simulink library "gm_dvbs2_stream_lib"  (R2025a)
settings: Solver=VariableStepAuto  StartTime=0.0  StopTime=10.0  RelTol=1e-3
undefined symbols (not defined in the file or in its folder): AXI4, Fs, gcbh, ip, Lite, soc
libraries: axiinterfacelib x6, xilinxsocsdrlib_internal x1, socsharedlib_internal x1
settings Model: Creator=daniel  LastModifiedBy=daniel

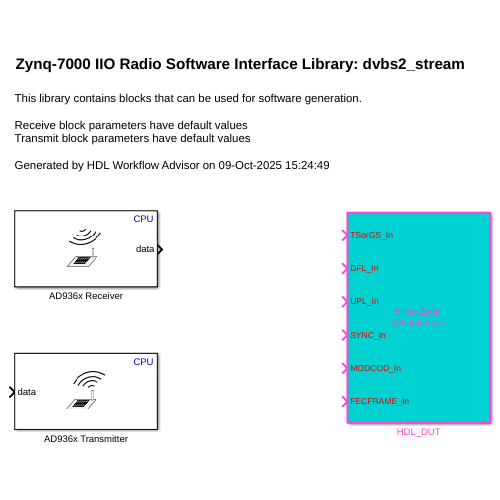
[thumbnail: Simulink's stored preview of the top-level diagram]
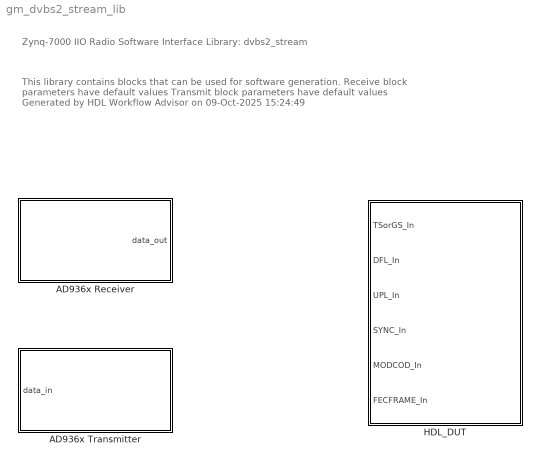
== system gm_dvbs2_stream_lib ==
  note: Zynq-7000 IIO Radio Software Interface Library: dvbs2_stream
  note: This library contains blocks that can be used for software generation.
      |
      | Receive block parameters have default values
      | Transmit block parameters have default values
      |
      | Generated by HDL Workflow Advisor on 09-Oct-2025 15:24:49
  AD936x Receiver : Subsystem  InitFcn=soc.blkcb.ad936xReadCb('InitFcn',gcbh);  mask(AD936x Data Read){SimulationInput=Zeros, IPAddress=192.168.3.2, CenterFrequencySource=Dialog, CenterFrequency=2400000000, GainSource=Dialog, Gain=10, BasebandSampleRate=1000000, EnableChannel1=on, EnableChannel2=off, OutputDataTypeStr=int16 (complex), SamplesPerFrame=20000, OverflowOutputPort=off, EnableBurstMode=off, NumFramesInBurst=2, UseCustomFilter=off, filtCoefficientSize=128, filtCoefficients=[-192 82 85 -215 228 -102 -110 290 -318 145 160 -426 471 -215 -238 633 -697 318 349 -923 1009 -457 -498 1309 -1423 640 693 -1812 1959 -876 -945 2458 -2647 1180 1268 -3290 3534 -1572 -1688 4375 -4698 2091 2247 -5836 6284 -2807 -3031 7918 -8588 3870 4225 -11182 12324 -5662 -6330 17255 -19735 9507 11312 -33568 43355 -25227 -42139 305542 305542 -42139 -25227 43355 -33568 11312 9507 -19735 17255 -6330 -5662 12324 -11182 4225 3870 -8588 7918 -3031 -2807 6284 -5836 2247 2091 -4698 4375 -1688 -1572 3534 -3290 1268 1180 -2647 2458 -945 -876 1959 -1812 693 640 -1423 1309 -498 -457 1009 -923 349 318 -697 633 -238 -215 471 -426 160 145 -318 290 -110 -102 228 -215 85 82 -192], filtDecimInterpFactor=4, filtGain=-12, filtPathRates=[737280000 11520000 3840000 1920000 960000 240000], filtRFBandwidth=18e6, filterConfigStruct=struct(), BypassUserLogic=off, EnableQuadratureCorrection=on, EnableRFDCCorrection=on, EnableBasebandDCCorrection=on, OverrideSampleTime=off, SampleTime=0.02, DataTimeout=Inf, BISTLoopbackMode=Disabled, BISTToneInject=Disabled, BISTSignalGen=PRBS, BISTToneFreq=Fs/32, BISTToneLevel=0}
      mask prompts: SimulationInput "Simulation input:"; IPAddress "Radio IP address:"; CenterFrequencySource "Source of center frequency:"; CenterFrequency "Center frequency (Hz):"; GainSource "Source of gain:"; Gain "Gain (dB):"; BasebandSampleRate "Baseband sample rate (Hz):"; EnableChannel1 "Enable Channel 1"; EnableChannel2 "Enable Channel 2"; OutputDataTypeStr "Output data type:"; SamplesPerFrame "Sample per frame:"; OverflowOutputPort "Enable output port for overflow indicator"; EnableBurstMode "Enable burst mode"; NumFramesInBurst "Frames in burst:"; UseCustomFilter "Use custom filter"; filtCoefficientSize "FIR coefficients size:"; filtCoefficients "FIR coefficients :"; filtDecimInterpFactor "FIR decimation/interpolation factor:"; filtGain "FIR gain (dB):"; filtPathRates "Filter path rates (Hz):"; filtRFBandwidth "Analog filter cutoff (Hz):"; filterConfigStruct "Filter config structure:"; BypassUserLogic "Bypass user logic"; EnableQuadratureCorrection "Enable quadrature correction"; EnableRFDCCorrection "Enable RF DC correction"; EnableBasebandDCCorrection "Enable baseband DC correction"; OverrideSampleTime "Override automatic sample time"; SampleTime "Sample time:"; DataTimeout "Data timeout (sec):"; BISTLoopbackMode "Loopback:"; BISTToneInject "Test signal injection:"; BISTSignalGen "Signal generator mode:"; BISTToneFreq "Tone frequency (Hz):"; BISTToneLevel "Tone level (dB):"
      mask help: soc:sdr:AD936xReadMaskText
      mask init:
      | soc.blkcb.ad936xReadCb('MaskInitFcn', gcbh);
      mask Help: helpview('soc', 'xilinxsoc_ad936x_data_read')
      mask TypeOptions SimulationInput: No data (configuration only) | Zeros | From connected IO
      mask Callback SimulationInput: soc.blkcb.ad936xReadCb('MaskParamCb',gcbh,'SimulationInput');
      mask TypeOptions IPAddress: Source Variant/From Connected IO/AD936x Receiver/IPAddress
      mask TypeOptions CenterFrequencySource: Source Variant/From Connected IO/AD936x Receiver/CenterFrequencySource | Source Variant/No Data/AD936x Receiver Config/CenterFrequencySource | Source Variant/Zeros/SimCodegen Variant/CODEGEN/AD936x Receiver/CenterFrequencySource
      mask Callback CenterFrequencySource: soc.blkcb.ad936xReadCb('MaskParamCb',gcbh,'CenterFrequencySource');
      mask TypeOptions CenterFrequency: Source Variant/From Connected IO/AD936x Receiver/CenterFrequency | Source Variant/No Data/AD936x Receiver Config/CenterFrequency | Source Variant/Zeros/SimCodegen Variant/CODEGEN/AD936x Receiver/CenterFrequency
      mask TypeOptions GainSource: Source Variant/From Connected IO/AD936x Receiver/GainSourceBlock | Source Variant/No Data/AD936x Receiver Config/GainSourceBlock | Source Variant/Zeros/SimCodegen Variant/CODEGEN/AD936x Receiver/GainSourceBlock
      mask Callback GainSource: soc.blkcb.ad936xReadCb('MaskParamCb',gcbh,'GainSource');
      mask TypeOptions Gain: Source Variant/From Connected IO/AD936x Receiver/Gain | Source Variant/No Data/AD936x Receiver Config/Gain | Source Variant/Zeros/SimCodegen Variant/CODEGEN/AD936x Receiver/Gain
      mask TypeOptions BasebandSampleRate: Source Variant/From Connected IO/AD936x Receiver/BasebandSampleRate | Source Variant/No Data/AD936x Receiver Config/BasebandSampleRate | Source Variant/Zeros/SimCodegen Variant/CODEGEN/AD936x Receiver/BasebandSampleRate
      mask TypeOptions OutputDataTypeStr: int16 (complex) | single (complex) | double (complex)
      mask TypeOptions OverflowOutputPort: Source Variant/From Connected IO/AD936x Receiver/OverflowOutputPort | Source Variant/Zeros/SimCodegen Variant/CODEGEN/AD936x Receiver/OverflowOutputPort
      mask TypeOptions EnableBurstMode: Source Variant/From Connected IO/AD936x Receiver/EnableBurstMode | Source Variant/Zeros/SimCodegen Variant/CODEGEN/AD936x Receiver/EnableBurstMode
      mask Callback EnableBurstMode: soc.blkcb.ad936xReadCb('MaskParamCb',gcbh,'EnableBurstMode');
      mask TypeOptions NumFramesInBurst: Source Variant/From Connected IO/AD936x Receiver/NumFramesInBurst | Source Variant/Zeros/SimCodegen Variant/CODEGEN/AD936x Receiver/NumFramesInBurst
      mask TypeOptions UseCustomFilter: Source Variant/From Connected IO/AD936x Receiver/UseCustomFilter | Source Variant/No Data/AD936x Receiver Config/UseCustomFilter | Source Variant/Zeros/SimCodegen Variant/CODEGEN/AD936x Receiver/UseCustomFilter
      mask Callback UseCustomFilter: soc.blkcb.ad936xReadCb('MaskParamCb',gcbh,'UseCustomFilter');
      mask TypeOptions filtCoefficientSize: Source Variant/From Connected IO/AD936x Receiver/filtCoefficientSize | Source Variant/No Data/AD936x Receiver Config/filtCoefficientSize | Source Variant/Zeros/SimCodegen Variant/CODEGEN/AD936x Receiver/filtCoefficientSize
      mask TypeOptions filtCoefficients: Source Variant/From Connected IO/AD936x Receiver/filtCoefficients | Source Variant/No Data/AD936x Receiver Config/filtCoefficients | Source Variant/Zeros/SimCodegen Variant/CODEGEN/AD936x Receiver/filtCoefficients
      mask TypeOptions filtDecimInterpFactor: Source Variant/From Connected IO/AD936x Receiver/filtDecimInterpFactor | Source Variant/No Data/AD936x Receiver Config/filtDecimInterpFactor | Source Variant/Zeros/SimCodegen Variant/CODEGEN/AD936x Receiver/filtDecimInterpFactor
      mask TypeOptions filtGain: Source Variant/From Connected IO/AD936x Receiver/filtGain | Source Variant/No Data/AD936x Receiver Config/filtGain | Source Variant/Zeros/SimCodegen Variant/CODEGEN/AD936x Receiver/filtGain
      mask TypeOptions filtPathRates: Source Variant/From Connected IO/AD936x Receiver/filtPathRates | Source Variant/No Data/AD936x Receiver Config/filtPathRates | Source Variant/Zeros/SimCodegen Variant/CODEGEN/AD936x Receiver/filtPathRates
      mask TypeOptions filtRFBandwidth: Source Variant/From Connected IO/AD936x Receiver/filtRFBandwidth | Source Variant/No Data/AD936x Receiver Config/filtRFBandwidth | Source Variant/Zeros/SimCodegen Variant/CODEGEN/AD936x Receiver/filtRFBandwidth
      mask TypeOptions filterConfigStruct: Source Variant/From Connected IO/AD936x Receiver/filterConfigStruct | Source Variant/No Data/AD936x Receiver Config/filterConfigStruct | Source Variant/Zeros/SimCodegen Variant/CODEGEN/AD936x Receiver/filterConfigStruct
      mask TypeOptions BypassUserLogic: Source Variant/From Connected IO/AD936x Receiver/BypassUserLogic | Source Variant/Zeros/SimCodegen Variant/CODEGEN/AD936x Receiver/BypassUserLogic
      mask TypeOptions EnableQuadratureCorrection: Source Variant/From Connected IO/AD936x Receiver/EnableQuadratureCorrection | Source Variant/No Data/AD936x Receiver Config/EnableQuadratureCorrection | Source Variant/Zeros/SimCodegen Variant/CODEGEN/AD936x Receiver/EnableQuadratureCorrection
      mask TypeOptions EnableRFDCCorrection: Source Variant/From Connected IO/AD936x Receiver/EnableRFDCCorrection | Source Variant/No Data/AD936x Receiver Config/EnableRFDCCorrection | Source Variant/Zeros/SimCodegen Variant/CODEGEN/AD936x Receiver/EnableRFDCCorrection
      mask TypeOptions EnableBasebandDCCorrection: Source Variant/From Connected IO/AD936x Receiver/EnableBasebandDCCorrection | Source Variant/No Data/AD936x Receiver Config/EnableBasebandDCCorrection | Source Variant/Zeros/SimCodegen Variant/CODEGEN/AD936x Receiver/EnableBasebandDCCorrection
      mask TypeOptions OverrideSampleTime: Source Variant/From Connected IO/AD936x Receiver/OverrideSampleTime | Source Variant/Zeros/SimCodegen Variant/CODEGEN/AD936x Receiver/OverrideSampleTime
      mask Callback OverrideSampleTime: soc.blkcb.ad936xReadCb('MaskParamCb',gcbh,'OverrideSampleTime');
      mask TypeOptions SampleTime: Source Variant/From Connected IO/AD936x Receiver/SampleTime | Source Variant/Zeros/SimCodegen Variant/CODEGEN/AD936x Receiver/SampleTime
      mask TypeOptions DataTimeout: Source Variant/From Connected IO/AD936x Receiver/DataTimeout | Source Variant/Zeros/SimCodegen Variant/CODEGEN/AD936x Receiver/DataTimeout
      mask TypeOptions BISTLoopbackMode: Source Variant/From Connected IO/AD936x Receiver/BISTLoopbackMode | Source Variant/Zeros/SimCodegen Variant/CODEGEN/AD936x Receiver/BISTLoopbackMode
      mask TypeOptions BISTToneInject: Source Variant/From Connected IO/AD936x Receiver/BISTToneInject | Source Variant/Zeros/SimCodegen Variant/CODEGEN/AD936x Receiver/BISTToneInject
      mask Callback BISTToneInject: soc.blkcb.ad936xReadCb('MaskParamCb',gcbh,'BISTToneInject');
      mask TypeOptions BISTSignalGen: Source Variant/From Connected IO/AD936x Receiver/BISTSignalGen | Source Variant/Zeros/SimCodegen Variant/CODEGEN/AD936x Receiver/BISTSignalGen
      mask Callback BISTSignalGen: soc.blkcb.ad936xReadCb('MaskParamCb',gcbh,'BISTSignalGen');
      mask TypeOptions BISTToneFreq: Source Variant/From Connected IO/AD936x Receiver/BISTToneFreq | Source Variant/Zeros/SimCodegen Variant/CODEGEN/AD936x Receiver/BISTToneFreq
      mask TypeOptions BISTToneLevel: Source Variant/From Connected IO/AD936x Receiver/BISTToneLevel | Source Variant/Zeros/SimCodegen Variant/CODEGEN/AD936x Receiver/BISTToneLevel
      mask DialogControl DescGroupVar Prompt: AD936x Data Read
      mask DialogControl MainTab Prompt: Main
      mask DialogControl RadioConnGrp Prompt: Radio Connection
      mask DialogControl InfoButton Prompt: Info
      mask DialogControl InfoButton Tooltip: Communicate with the attached radio to test connectivity and to determine quantized radio configuration values.
      mask DialogControl InfoButton Callback: soc.blkcb.ad936xReadCb('InfoButtonCb',gcbh);
      mask DialogControl RadioPropGrp Prompt: Radio Properties
      mask DialogControl DataGrp Prompt: Data
      mask DialogControl FilterTab Prompt: Filter
      mask DialogControl CustomFilterConfigGrp Prompt: Custom Filter Configuration
      mask DialogControl FilterWizardButton Prompt: Launch filter wizard
      mask DialogControl FilterWizardButton Callback: soc.blkcb.ad936xReadCb('FilterWizardButtonCb',gcbh);
      mask DialogControl AdvancedTab Prompt: Advanced
      mask DialogControl AdvRadioPropGrp Prompt: Radio Properties
      mask DialogControl AdvDataGrp Prompt: Data
      mask DialogControl BISTConfigGrp Prompt: Built-In Self-Test Configuration
      mask Display:
      | color('blue'); text(0.98,0.93,'CPU','horizontalAlignment','right','texmode','on'); color('black');
      | 
      | port_label('output', 1, 'data');
  AD936x Transmitter : Subsystem  InitFcn=soc.blkcb.ad936xWriteCb('InitFcn',gcbh);  mask(AD936x Data Write){SimulationOutput=Terminator, IPAddress=192.168.3.2, CenterFrequencySource=Dialog, CenterFrequency=2400000000, GainSource=Dialog, Gain=-10, BasebandSampleRate=1000000, EnableChannel1=on, EnableChannel2=off, UnderflowOutputPort=off, UseCustomFilter=off, filtCoefficientSize=128, filtCoefficients=[-192 82 85 -215 228 -102 -110 290 -318 145 160 -426 471 -215 -238 633 -697 318 349 -923 1009 -457 -498 1309 -1423 640 693 -1812 1959 -876 -945 2458 -2647 1180 1268 -3290 3534 -1572 -1688 4375 -4698 2091 2247 -5836 6284 -2807 -3031 7918 -8588 3870 4225 -11182 12324 -5662 -6330 17255 -19735 9507 11312 -33568 43355 -25227 -42139 305542 305542 -42139 -25227 43355 -33568 11312 9507 -19735 17255 -6330 -5662 12324 -11182 4225 3870 -8588 7918 -3031 -2807 6284 -5836 2247 2091 -4698 4375 -1688 -1572 3534 -3290 1268 1180 -2647 2458 -945 -876 1959 -1812 693 640 -1423 1309 -498 -457 1009 -923 349 318 -697 633 -238 -215 471 -426 160 145 -318 290 -110 -102 228 -215 85 82 -192], filtDecimInterpFactor=4, filtGain=-12, filtPathRates=[737280000 11520000 3840000 1920000 960000 240000], filtRFBandwidth=18000000, filterConfigStruct=struct(), BypassUserLogic=off, DataSourceSelect=Input Port, DDSTone1Freq=5000, DDSTone2Freq=10000, DDSTone1Scale=0.5, DDSTone2Scale=0.25, DataTimeout=Inf, BISTLoopbackMode=Disabled, BISTToneInject=Disabled, BISTSignalGen=PRBS, BISTToneFreq=Fs/32, BISTToneLevel=0}
      mask prompts: SimulationOutput "Simulation output:"; IPAddress "Radio IP address:"; CenterFrequencySource "Source of center frequency:"; CenterFrequency "Center frequency (Hz):"; GainSource "Source of gain:"; Gain "Gain (dB):"; BasebandSampleRate "Baseband sample rate (Hz):"; EnableChannel1 "Enable Channel 1"; EnableChannel2 "Enable Channel 2"; UnderflowOutputPort "Enable output port for underflow indicator"; UseCustomFilter "Use custom filter"; filtCoefficientSize "FIR coefficients size:"; filtCoefficients "FIR coefficients :"; filtDecimInterpFactor "FIR decimation/interpolation factor:"; filtGain "FIR gain (dB):"; filtPathRates "Filter path rates (Hz):"; filtRFBandwidth "Analog filter cutoff (Hz):"; filterConfigStruct "Filter config structure:"; BypassUserLogic "Bypass user logic"; DataSourceSelect "Data source select:"; DDSTone1Freq "Tone 1 Frequency (Hz):"; DDSTone2Freq "Tone 2 Frequency (Hz):"; DDSTone1Scale "Tone 1 Scale [0-1]:"; DDSTone2Scale "Tone 2 Scale [0-1]:"; DataTimeout "Data timeout (sec):"; BISTLoopbackMode "Loopback:"; BISTToneInject "Test signal injection:"; BISTSignalGen "Signal generator mode:"; BISTToneFreq "Tone frequency (Hz):"; BISTToneLevel "Tone level (dB):"
      mask help: soc:sdr:AD936xWriteMaskText
      mask init:
      | soc.blkcb.ad936xWriteCb('MaskInitFcn', gcbh);
      mask Help: helpview('soc', 'xilinxsoc_ad936x_data_write')
      mask TypeOptions SimulationOutput: No data (configuration only) | Terminator | To connected IO
      mask Callback SimulationOutput: soc.blkcb.ad936xWriteCb('MaskParamCb',gcbh,'SimulationOutput');
      mask TypeOptions IPAddress: Sink Variant/To Connected IO/AD936x Transmitter/IPAddress
      mask TypeOptions CenterFrequencySource: Sink Variant/No Data/AD936x Transmitter Config/CenterFrequencySource | Sink Variant/Terminator/SimCodegen Variant/CODEGEN/AD936x Transmitter/CenterFrequencySource | Sink Variant/To Connected IO/AD936x Transmitter/CenterFrequencySource
      mask Callback CenterFrequencySource: soc.blkcb.ad936xWriteCb('MaskParamCb',gcbh,'CenterFrequencySource');
      mask TypeOptions CenterFrequency: Sink Variant/No Data/AD936x Transmitter Config/CenterFrequency | Sink Variant/Terminator/SimCodegen Variant/CODEGEN/AD936x Transmitter/CenterFrequency | Sink Variant/To Connected IO/AD936x Transmitter/CenterFrequency
      mask TypeOptions GainSource: Sink Variant/No Data/AD936x Transmitter Config/GainSource | Sink Variant/Terminator/SimCodegen Variant/CODEGEN/AD936x Transmitter/GainSource | Sink Variant/To Connected IO/AD936x Transmitter/GainSource
      mask Callback GainSource: soc.blkcb.ad936xWriteCb('MaskParamCb',gcbh,'GainSource');
      mask TypeOptions Gain: Sink Variant/No Data/AD936x Transmitter Config/Gain | Sink Variant/Terminator/SimCodegen Variant/CODEGEN/AD936x Transmitter/Gain | Sink Variant/To Connected IO/AD936x Transmitter/Gain
      mask TypeOptions BasebandSampleRate: Sink Variant/No Data/AD936x Transmitter Config/BasebandSampleRate | Sink Variant/Terminator/SimCodegen Variant/CODEGEN/AD936x Transmitter/BasebandSampleRate | Sink Variant/To Connected IO/AD936x Transmitter/BasebandSampleRate
      mask TypeOptions UnderflowOutputPort: Sink Variant/Terminator/SimCodegen Variant/CODEGEN/AD936x Transmitter/UnderflowOutputPort | Sink Variant/To Connected IO/AD936x Transmitter/UnderflowOutputPort
      mask TypeOptions UseCustomFilter: Sink Variant/No Data/AD936x Transmitter Config/UseCustomFilter | Sink Variant/Terminator/SimCodegen Variant/CODEGEN/AD936x Transmitter/UseCustomFilter | Sink Variant/To Connected IO/AD936x Transmitter/UseCustomFilter
      mask Callback UseCustomFilter: soc.blkcb.ad936xWriteCb('MaskParamCb',gcbh,'UseCustomFilter');
      mask TypeOptions filtCoefficientSize: Sink Variant/No Data/AD936x Transmitter Config/filtCoefficientSize | Sink Variant/Terminator/SimCodegen Variant/CODEGEN/AD936x Transmitter/filtCoefficientSize | Sink Variant/To Connected IO/AD936x Transmitter/filtCoefficientSize
      mask TypeOptions filtCoefficients: Sink Variant/No Data/AD936x Transmitter Config/filtCoefficients | Sink Variant/Terminator/SimCodegen Variant/CODEGEN/AD936x Transmitter/filtCoefficients | Sink Variant/To Connected IO/AD936x Transmitter/filtCoefficients
      mask TypeOptions filtDecimInterpFactor: Sink Variant/No Data/AD936x Transmitter Config/filtDecimInterpFactor | Sink Variant/Terminator/SimCodegen Variant/CODEGEN/AD936x Transmitter/filtDecimInterpFactor | Sink Variant/To Connected IO/AD936x Transmitter/filtDecimInterpFactor
      mask TypeOptions filtGain: Sink Variant/No Data/AD936x Transmitter Config/filtGain | Sink Variant/Terminator/SimCodegen Variant/CODEGEN/AD936x Transmitter/filtGain | Sink Variant/To Connected IO/AD936x Transmitter/filtGain
      mask TypeOptions filtPathRates: Sink Variant/No Data/AD936x Transmitter Config/filtPathRates | Sink Variant/Terminator/SimCodegen Variant/CODEGEN/AD936x Transmitter/filtPathRates | Sink Variant/To Connected IO/AD936x Transmitter/filtPathRates
      mask TypeOptions filtRFBandwidth: Sink Variant/No Data/AD936x Transmitter Config/filtRFBandwidth | Sink Variant/Terminator/SimCodegen Variant/CODEGEN/AD936x Transmitter/filtRFBandwidth | Sink Variant/To Connected IO/AD936x Transmitter/filtRFBandwidth
      mask TypeOptions filterConfigStruct: Sink Variant/No Data/AD936x Transmitter Config/filterConfigStruct | Sink Variant/Terminator/SimCodegen Variant/CODEGEN/AD936x Transmitter/filterConfigStruct | Sink Variant/To Connected IO/AD936x Transmitter/filterConfigStruct
      mask TypeOptions BypassUserLogic: Sink Variant/Terminator/SimCodegen Variant/CODEGEN/AD936x Transmitter/BypassUserLogic | Sink Variant/To Connected IO/AD936x Transmitter/BypassUserLogic
      mask TypeOptions DataSourceSelect: Sink Variant/No Data/AD936x Transmitter Config/DataSourceSelect | Sink Variant/Terminator/SimCodegen Variant/CODEGEN/AD936x Transmitter/DataSourceSelect | Sink Variant/To Connected IO/AD936x Transmitter/DataSourceSelect
      mask Callback DataSourceSelect: soc.blkcb.ad936xWriteCb('MaskParamCb',gcbh,'DataSourceSelect');
      mask TypeOptions DDSTone1Freq: Sink Variant/No Data/AD936x Transmitter Config/DDSTone1Freq | Sink Variant/Terminator/SimCodegen Variant/CODEGEN/AD936x Transmitter/DDSTone1Freq | Sink Variant/To Connected IO/AD936x Transmitter/DDSTone1Freq
      mask TypeOptions DDSTone2Freq: Sink Variant/No Data/AD936x Transmitter Config/DDSTone2Freq | Sink Variant/Terminator/SimCodegen Variant/CODEGEN/AD936x Transmitter/DDSTone2Freq | Sink Variant/To Connected IO/AD936x Transmitter/DDSTone2Freq
      mask TypeOptions DDSTone1Scale: Sink Variant/No Data/AD936x Transmitter Config/DDSTone1Scale | Sink Variant/Terminator/SimCodegen Variant/CODEGEN/AD936x Transmitter/DDSTone1Scale | Sink Variant/To Connected IO/AD936x Transmitter/DDSTone1Scale
      mask TypeOptions DDSTone2Scale: Sink Variant/No Data/AD936x Transmitter Config/DDSTone2Scale | Sink Variant/Terminator/SimCodegen Variant/CODEGEN/AD936x Transmitter/DDSTone2Scale | Sink Variant/To Connected IO/AD936x Transmitter/DDSTone2Scale
      mask TypeOptions DataTimeout: Sink Variant/Terminator/SimCodegen Variant/CODEGEN/AD936x Transmitter/DataTimeout | Sink Variant/To Connected IO/AD936x Transmitter/DataTimeout
      mask TypeOptions BISTLoopbackMode: Sink Variant/Terminator/SimCodegen Variant/CODEGEN/AD936x Transmitter/BISTLoopbackMode | Sink Variant/To Connected IO/AD936x Transmitter/BISTLoopbackMode
      mask TypeOptions BISTToneInject: Sink Variant/Terminator/SimCodegen Variant/CODEGEN/AD936x Transmitter/BISTToneInject | Sink Variant/To Connected IO/AD936x Transmitter/BISTToneInject
      mask Callback BISTToneInject: soc.blkcb.ad936xWriteCb('MaskParamCb',gcbh,'BISTToneInject');
      mask TypeOptions BISTSignalGen: Sink Variant/Terminator/SimCodegen Variant/CODEGEN/AD936x Transmitter/BISTSignalGen | Sink Variant/To Connected IO/AD936x Transmitter/BISTSignalGen
      mask Callback BISTSignalGen: soc.blkcb.ad936xWriteCb('MaskParamCb',gcbh,'BISTSignalGen');
      mask TypeOptions BISTToneFreq: Sink Variant/Terminator/SimCodegen Variant/CODEGEN/AD936x Transmitter/BISTToneFreq | Sink Variant/To Connected IO/AD936x Transmitter/BISTToneFreq
      mask TypeOptions BISTToneLevel: Sink Variant/Terminator/SimCodegen Variant/CODEGEN/AD936x Transmitter/BISTToneLevel | Sink Variant/To Connected IO/AD936x Transmitter/BISTToneLevel
      mask DialogControl DescGroupVar Prompt: AD936x Data Write
      mask DialogControl MainTab Prompt: Main
      mask DialogControl RadioConnGrp Prompt: Radio Connection
      mask DialogControl InfoButton Prompt: Info
      mask DialogControl InfoButton Callback: soc.blkcb.ad936xWriteCb('InfoButtonCb',gcbh);
      mask DialogControl RadioPropGrp Prompt: Radio Properties
      mask DialogControl DataGrp Prompt: Data
      mask DialogControl FilterTab Prompt: Filter
      mask DialogControl CustomFilterConfigGrp Prompt: Custom Filter Configuration
      mask DialogControl FilterWizardButton Prompt: Launch filter wizard
      mask DialogControl FilterWizardButton Callback: soc.blkcb.ad936xWriteCb('FilterWizardButtonCb',gcbh);
      mask DialogControl AdvancedTab Prompt: Advanced
      mask DialogControl AdvRadioPropGrp Prompt: Radio Properties
      mask DialogControl AdvDataGrp Prompt: Data
      mask DialogControl BISTConfigGrp Prompt: Built-In Self-Test Configuration
      mask Display:
      | color('blue'); text(0.98,0.93,'CPU','horizontalAlignment','right','texmode','on'); color('black');
      | port_label('input', 1, 'data');
  HDL_DUT : Subsystem  TreatAsAtomicUnit=on  mask(AXI4-Lite/AXI4 Interface){}
      mask help:
      | This is an automatically generated subsystem block.
      | This contains the AXI interface blocks that communicate with the DVBS2_Stream_ip_v0_1 IPCore generated from dvbs2_stream/HDL_DUT subsystem.
      mask Display: disp(sprintf('Xilinx Zynq \nAXI Interface'));

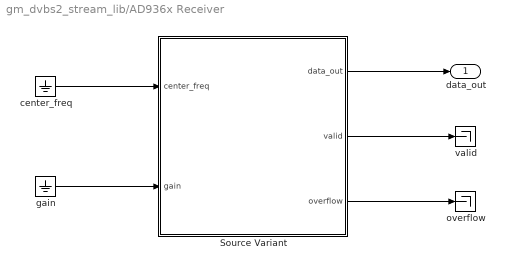
== system gm_dvbs2_stream_lib/AD936x Receiver ==
  Source Variant : Subsystem  Variant=on  VariantControlMode=label  LabelModeActiveChoice=Zeros
  center_freq : Ground
  gain : Ground
  overflow : Terminator
  valid : Terminator
  data_out : Outport
  wires:
  Source Variant/2(valid) -> valid/1
  Source Variant/3(overflow) -> overflow/1
  gain/1 -> Source Variant/2(gain)
  center_freq/1 -> Source Variant/1(center_freq)
  Source Variant/1(data_out) -> data_out/1

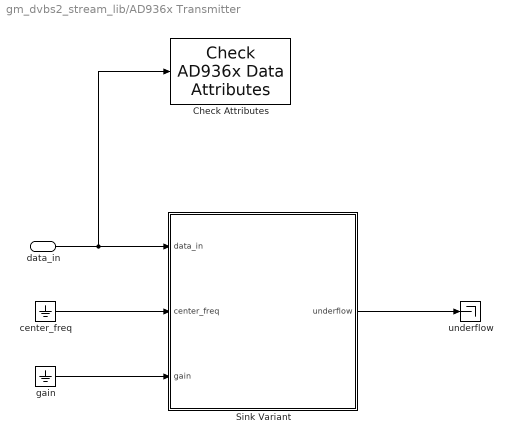
== system gm_dvbs2_stream_lib/AD936x Transmitter ==
  data_in : Inport
  Check Attributes : xilinxsocsdrlib_internal/Check AD936x Data Attributes  dt_int16=on  dt_uint32=off  dt_single=on  dt_double=on  channelnum=1  stype=complex  ptype=gm_dvbs2_stream_lib/AD936x Transmitter
  Sink Variant : Subsystem  Variant=on  VariantControlMode=label  LabelModeActiveChoice=Terminator
  center_freq : Ground
  gain : Ground
  underflow : Terminator
  wires:
  Sink Variant/1(underflow) -> underflow/1
  gain/1 -> Sink Variant/3(gain)
  data_in/1 -> Sink Variant/1(data_in), Check Attributes/1
  center_freq/1 -> Sink Variant/2(center_freq)

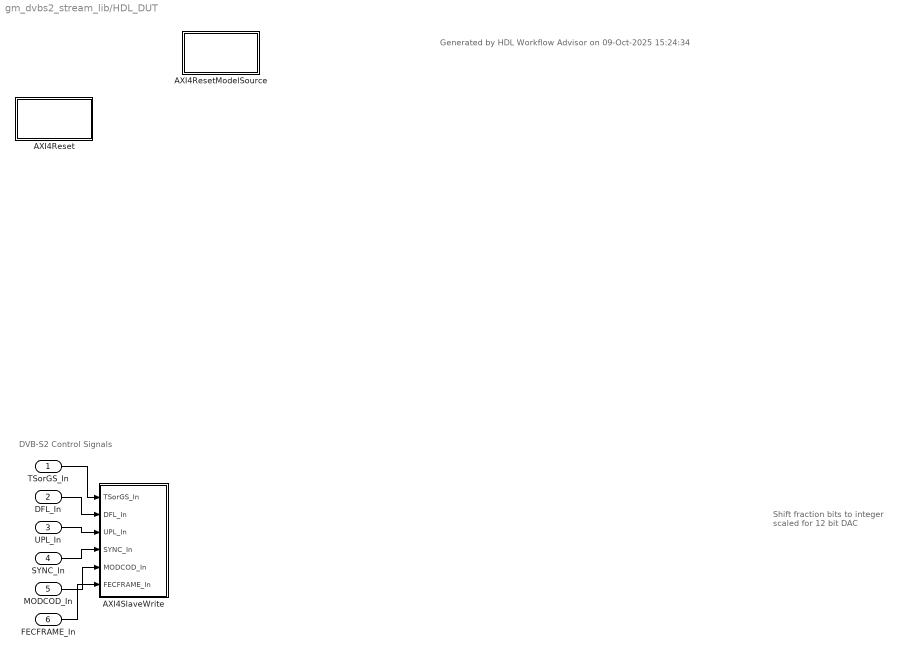
== system gm_dvbs2_stream_lib/HDL_DUT ==
  note: Generated by HDL Workflow Advisor on 09-Oct-2025 15:24:34
  note: Shift fraction bits to integer scaled for 12 bit DAC
  note: DVB-S2 Control Signals
  TSorGS_In : Inport
  DFL_In : Inport  Port=2
  UPL_In : Inport  Port=3
  SYNC_In : Inport  Port=4
  MODCOD_In : Inport  Port=5
  FECFRAME_In : Inport  Port=6
  AXI4Reset : Subsystem  mask(System Start){ShowInLibBrowser=0}
      mask prompts: ShowInLibBrowser "Simulink:masks:CustCodeMaskParam1_MP"
      settings: CopyFcn=cccopyfcn(gcb)  OpenFcn=ccopenfcn('System Start Function')
      mask Help: eval('feval(''rtwprivate'',''rtwhelpview'',''rtw_sys_start_block'')');
      mask Display: disp('System\nStart');
  AXI4ResetModelSource : Subsystem  mask(Model Source){ShowInLibBrowser=0}
      mask prompts: ShowInLibBrowser "Simulink:masks:CustCodeMaskParam1_MP"
      settings: CopyFcn=cccopyfcn(gcb)  OpenFcn=ccopenfcn('Model Source')
      mask Help: eval('feval(''rtwprivate'',''rtwhelpview'',''rtw_model_source_block'')');
      mask Display: disp('Model\nSource');
  AXI4SlaveWrite : Subsystem  Priority=1
  wires:
  FECFRAME_In/1 -> AXI4SlaveWrite/6(FECFRAME_In)
  MODCOD_In/1 -> AXI4SlaveWrite/5(MODCOD_In)
  SYNC_In/1 -> AXI4SlaveWrite/4(SYNC_In)
  UPL_In/1 -> AXI4SlaveWrite/3(UPL_In)
  DFL_In/1 -> AXI4SlaveWrite/2(DFL_In)
  TSorGS_In/1 -> AXI4SlaveWrite/1(TSorGS_In)

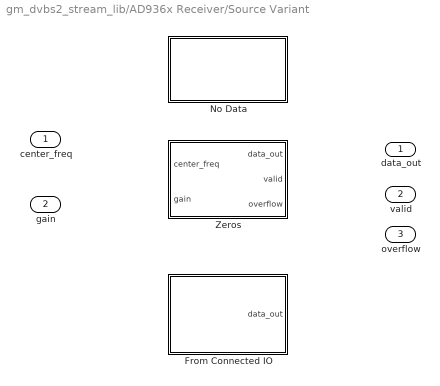
== system gm_dvbs2_stream_lib/AD936x Receiver/Source Variant ==
  center_freq : Inport
  gain : Inport  Port=2
  From Connected IO : Subsystem  VariantControl=FromConnectedIO
  No Data : Subsystem  VariantControl=NoData
  Zeros : Subsystem  VariantControl=Zeros
  data_out : Outport
  valid : Outport  Port=2
  overflow : Outport  Port=3

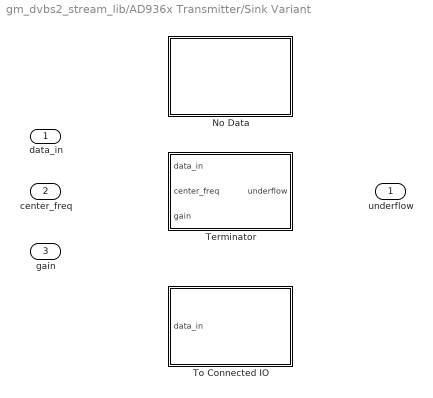
== system gm_dvbs2_stream_lib/AD936x Transmitter/Sink Variant ==
  data_in : Inport
  center_freq : Inport  Port=2
  gain : Inport  Port=3
  No Data : Subsystem  VariantControl=NoData
  Terminator : Subsystem  VariantControl=Terminator
  To Connected IO : Subsystem  VariantControl=ToConnectedIO
  underflow : Outport

== system gm_dvbs2_stream_lib/HDL_DUT/AXI4Reset ==

== system gm_dvbs2_stream_lib/HDL_DUT/AXI4ResetModelSource ==

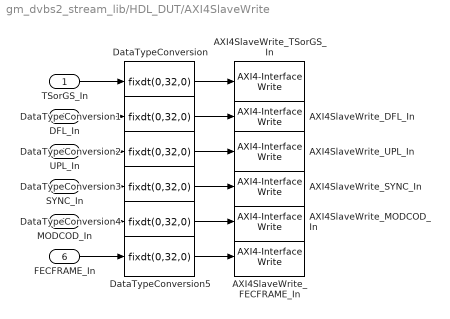
== system gm_dvbs2_stream_lib/HDL_DUT/AXI4SlaveWrite ==
  TSorGS_In : Inport
  DFL_In : Inport  Port=2
  UPL_In : Inport  Port=3
  SYNC_In : Inport  Port=4
  MODCOD_In : Inport  Port=5
  FECFRAME_In : Inport  Port=6
  AXI4SlaveWrite_DFL_In : axiinterfacelib/AXI4-Interface Write  Priority=3  AXIInterfaceType=AXI4-Lite  DeviceName=/dev/mwipcore  RegisterOffset=hex2dec('104')  blockPlatform=ZYNQ  SimulateUsing=Interpreted execution
  AXI4SlaveWrite_FECFRAME_In : axiinterfacelib/AXI4-Interface Write  Priority=7  AXIInterfaceType=AXI4-Lite  DeviceName=/dev/mwipcore  RegisterOffset=hex2dec('114')  blockPlatform=ZYNQ  SimulateUsing=Interpreted execution
  AXI4SlaveWrite_MODCOD_In : axiinterfacelib/AXI4-Interface Write  Priority=6  AXIInterfaceType=AXI4-Lite  DeviceName=/dev/mwipcore  RegisterOffset=hex2dec('110')  blockPlatform=ZYNQ  SimulateUsing=Interpreted execution
  AXI4SlaveWrite_SYNC_In : axiinterfacelib/AXI4-Interface Write  Priority=5  AXIInterfaceType=AXI4-Lite  DeviceName=/dev/mwipcore  RegisterOffset=hex2dec('10C')  blockPlatform=ZYNQ  SimulateUsing=Interpreted execution
  AXI4SlaveWrite_TSorGS_In : axiinterfacelib/AXI4-Interface Write  Priority=2  AXIInterfaceType=AXI4-Lite  DeviceName=/dev/mwipcore  RegisterOffset=hex2dec('100')  blockPlatform=ZYNQ  SimulateUsing=Interpreted execution
  AXI4SlaveWrite_UPL_In : axiinterfacelib/AXI4-Interface Write  Priority=4  AXIInterfaceType=AXI4-Lite  DeviceName=/dev/mwipcore  RegisterOffset=hex2dec('108')  blockPlatform=ZYNQ  SimulateUsing=Interpreted execution
  DataTypeConversion{,1..5} (6 alike) : DataTypeConversion  OutDataTypeStr=fixdt(0,32,0)  ConvertRealWorld=Stored Integer (SI)  SaturateOnIntegerOverflow=off  RndMeth=Floor
  wires:
  DFL_In/1 -> DataTypeConversion1/1
  SYNC_In/1 -> DataTypeConversion3/1
  DataTypeConversion5/1 -> AXI4SlaveWrite_FECFRAME_In/1
  DataTypeConversion1/1 -> AXI4SlaveWrite_DFL_In/1
  DataTypeConversion3/1 -> AXI4SlaveWrite_SYNC_In/1
  MODCOD_In/1 -> DataTypeConversion4/1
  FECFRAME_In/1 -> DataTypeConversion5/1
  DataTypeConversion4/1 -> AXI4SlaveWrite_MODCOD_In/1
  DataTypeConversion2/1 -> AXI4SlaveWrite_UPL_In/1
  UPL_In/1 -> DataTypeConversion2/1
  TSorGS_In/1 -> DataTypeConversion/1
  DataTypeConversion/1 -> AXI4SlaveWrite_TSorGS_In/1

== system gm_dvbs2_stream_lib/AD936x Receiver/Source Variant/From Connected IO ==
  AD936x Receiver : MATLABSystem  System=comm.SDRRxAD936x  IPAddress=192.168.3.2  uri=ip:10.0.0.200  CenterFrequencySource=Dialog  CenterFrequency=CenterFrequency  GainSource=AGC Slow Attack  GainSourceBlock=Dialog  Gain=Gain  ChannelMapping=1  BasebandSampleRate=BasebandSampleRate  OutputDataType=int16  SamplesPerFrame=20000  OverflowOutputPort=off  EnableBurstMode=off  NumFramesInBurst=NumFramesInBurst  ShowAdvancedProperties=off  UseCustomFilter=off  filtPathRates=filtPathRates  filtCoefficients=filtCoefficients  filtCoefficientSize=filtCoefficientSize  filtDecimInterpFactor=filtDecimInterpFactor  filtGain=filtGain  filtRFBandwidth=filtRFBandwidth  filterConfigStruct=filterConfigStruct  BypassUserLogic=off  EnableQuadratureCorrection=on  EnableRFDCCorrection=on  EnableBasebandDCCorrection=on  OverrideSampleTime=off  SampleTime=SampleTime  DataTimeout=DataTimeout  ENSMPinControlMode=None  BISTLoopbackMode=Disabled  BISTToneInject=Disabled  BISTSignalGen=PRBS  BISTToneFreq=Fs/32  BISTToneLevel=0
      mask Type: comm.SDRRxAD936x
  data_out : Outport
  wires:
  AD936x Receiver/1 -> data_out/1

== system gm_dvbs2_stream_lib/AD936x Receiver/Source Variant/No Data ==
  AD936x Receiver Config : MATLABSystem  InitFcn=|  System=comm.internal.SDRRxZC706FMC234RFSL  uri=ip:10.0.0.200  CenterFrequencySource=Dialog  CenterFrequency=CenterFrequency  GainSource=AGC Slow Attack  GainSourceBlock=Dialog  Gain=Gain  ChannelMapping=1  BasebandSampleRate=BasebandSampleRate  ShowAdvancedProperties=off  DataTimeout=Inf  EnableQuadratureCorrection=on  EnableRFDCCorrection=on  EnableBasebandDCCorrection=on  UseCustomFilter=off  filtPathRates=filtPathRates  filtCoefficients=filtCoefficients  filtCoefficientSize=filtCoefficientSize  filtDecimInterpFactor=filtDecimInterpFactor  filtGain=filtGain  filtRFBandwidth=filtRFBandwidth  filterConfigStruct=filterConfigStruct
      | sdr.internal.registerRFBlocks(gcb);
      | sdr.internal.validateRequireTpToolsAndAddToPath(gcb);
      mask Type: comm.internal.SDRRxZC706FMC234RFSL

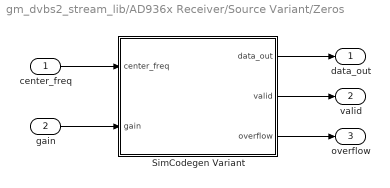
== system gm_dvbs2_stream_lib/AD936x Receiver/Source Variant/Zeros ==
  center_freq : Inport
  gain : Inport  Port=2
  SimCodegen Variant : Subsystem  Variant=on  VariantControlMode=sim codegen switching
  data_out : Outport
  valid : Outport  Port=2
  overflow : Outport  Port=3
  wires:
  SimCodegen Variant/3(overflow) -> overflow/1
  SimCodegen Variant/2(valid) -> valid/1
  SimCodegen Variant/1(data_out) -> data_out/1
  gain/1 -> SimCodegen Variant/2(gain)
  center_freq/1 -> SimCodegen Variant/1(center_freq)

== system gm_dvbs2_stream_lib/AD936x Transmitter/Sink Variant/No Data ==
  AD936x Transmitter Config : MATLABSystem  InitFcn=|  System=comm.internal.SDRTxZC706FMC234RFSL  IPAddress=192.168.3.2  uri=ip:10.0.0.200  CenterFrequencySource=Dialog  CenterFrequency=CenterFrequency  GainSource=Dialog  Gain=Gain  ChannelMapping=1  BasebandSampleRate=BasebandSampleRate  ShowAdvancedProperties=on  DataSourceSelect=Input Port  DDSTone1Freq=DDSTone1Freq  DDSTone2Freq=DDSTone2Freq  DDSTone1Scale=DDSTone1Scale  DDSTone2Scale=DDSTone2Scale  DataTimeout=Inf  UseCustomFilter=off  filtPathRates=filtPathRates  filtCoefficients=filtCoefficients  filtCoefficientSize=filtCoefficientSize  filtDecimInterpFactor=filtDecimInterpFactor  filtGain=filtGain  filtRFBandwidth=filtRFBandwidth  filterConfigStruct=filterConfigStruct
      | sdr.internal.registerRFBlocks(gcb);
      | sdr.internal.validateRequireTpToolsAndAddToPath(gcb);
      mask Type: comm.internal.SDRTxZC706FMC234RFSL

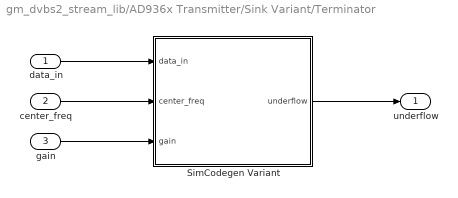
== system gm_dvbs2_stream_lib/AD936x Transmitter/Sink Variant/Terminator ==
  data_in : Inport
  center_freq : Inport  Port=2
  gain : Inport  Port=3
  SimCodegen Variant : Subsystem  Variant=on  VariantControlMode=sim codegen switching
  underflow : Outport
  wires:
  SimCodegen Variant/1(underflow) -> underflow/1
  gain/1 -> SimCodegen Variant/3(gain)
  center_freq/1 -> SimCodegen Variant/2(center_freq)
  data_in/1 -> SimCodegen Variant/1(data_in)

== system gm_dvbs2_stream_lib/AD936x Transmitter/Sink Variant/To Connected IO ==
  data_in : Inport
  AD936x Transmitter : MATLABSystem  System=comm.SDRTxAD936x  IPAddress=192.168.3.2  uri=ip:10.0.0.200  CenterFrequencySource=Dialog  CenterFrequency=CenterFrequency  GainSource=Dialog  Gain=Gain  ChannelMapping=1  BasebandSampleRate=BasebandSampleRate  UnderflowOutputPort=off  ShowAdvancedProperties=off  UseCustomFilter=off  filtPathRates=filtPathRates  filtCoefficients=filtCoefficients  filtCoefficientSize=filtCoefficientSize  filtDecimInterpFactor=filtDecimInterpFactor  filtGain=filtGain  filtRFBandwidth=filtRFBandwidth  filterConfigStruct=filterConfigStruct  BypassUserLogic=off  DataSourceSelect=Input Port  DDSTone1Freq=DDSTone1Freq  DDSTone2Freq=DDSTone2Freq  DDSTone1Scale=DDSTone1Scale  DDSTone2Scale=DDSTone2Scale  DataTimeout=DataTimeout  ENSMPinControlMode=None  BISTLoopbackMode=Disabled  BISTToneInject=Disabled  BISTSignalGen=PRBS  BISTToneFreq=Fs/32  BISTToneLevel=0
      mask Type: comm.SDRTxAD936x
  wires:
  data_in/1 -> AD936x Transmitter/1

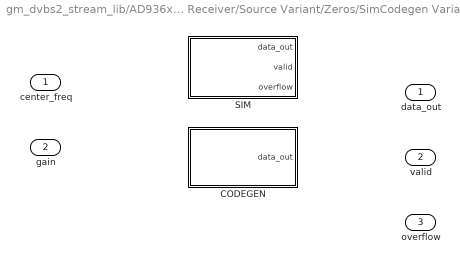
== system gm_dvbs2_stream_lib/AD936x Receiver/Source Variant/Zeros/SimCodegen Variant ==
  center_freq : Inport
  gain : Inport  Port=2
  CODEGEN : Subsystem  VariantControl=(codegen)
  SIM : Subsystem  VariantControl=(sim)
  data_out : Outport
  valid : Outport  Port=2
  overflow : Outport  Port=3

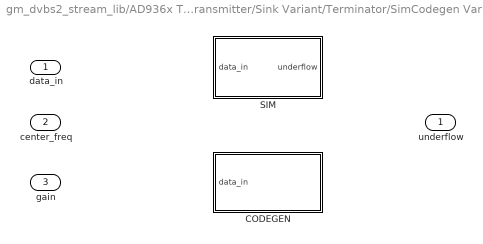
== system gm_dvbs2_stream_lib/AD936x Transmitter/Sink Variant/Terminator/SimCodegen Variant ==
  data_in : Inport
  center_freq : Inport  Port=2
  gain : Inport  Port=3
  CODEGEN : Subsystem  VariantControl=(codegen)
  SIM : Subsystem  VariantControl=(sim)
  underflow : Outport

== system gm_dvbs2_stream_lib/AD936x Receiver/Source Variant/Zeros/SimCodegen Variant/CODEGEN ==
  AD936x Receiver : MATLABSystem  System=comm.SDRRxAD936x  IPAddress=192.168.3.2  uri=ip:10.0.0.200  CenterFrequencySource=Dialog  CenterFrequency=CenterFrequency  GainSource=AGC Slow Attack  GainSourceBlock=Dialog  Gain=Gain  ChannelMapping=1  BasebandSampleRate=BasebandSampleRate  OutputDataType=int16  SamplesPerFrame=20000  OverflowOutputPort=off  EnableBurstMode=off  NumFramesInBurst=NumFramesInBurst  ShowAdvancedProperties=off  UseCustomFilter=off  filtPathRates=filtPathRates  filtCoefficients=filtCoefficients  filtCoefficientSize=filtCoefficientSize  filtDecimInterpFactor=filtDecimInterpFactor  filtGain=filtGain  filtRFBandwidth=filtRFBandwidth  filterConfigStruct=filterConfigStruct  BypassUserLogic=off  EnableQuadratureCorrection=on  EnableRFDCCorrection=on  EnableBasebandDCCorrection=on  OverrideSampleTime=off  SampleTime=SampleTime  DataTimeout=DataTimeout  ENSMPinControlMode=None  BISTLoopbackMode=Disabled  BISTToneInject=Disabled  BISTSignalGen=PRBS  BISTToneFreq=Fs/32  BISTToneLevel=0
      mask Type: comm.SDRRxAD936x
  data_out : Outport
  wires:
  AD936x Receiver/1 -> data_out/1

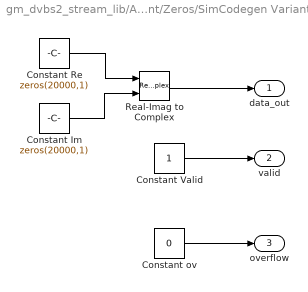
== system gm_dvbs2_stream_lib/AD936x Receiver/Source Variant/Zeros/SimCodegen Variant/SIM ==
  Constant Im : Constant  Value=zeros(20000,1)  VectorParams1D=off  OutDataTypeStr=int16  SampleTime=20000/1000000
  Constant Re : Constant  Value=zeros(20000,1)  VectorParams1D=off  OutDataTypeStr=int16  SampleTime=20000/1000000
  Constant Valid : Constant  OutDataTypeStr=boolean  SampleTime=20000/1000000
  Constant ov : Constant  Value=0  OutDataTypeStr=boolean  SampleTime=20000/1000000
  Real-Imag to Complex : RealImagToComplex
  data_out : Outport
  valid : Outport  Port=2
  overflow : Outport  Port=3
  wires:
  Constant Valid/1 -> valid/1
  Constant ov/1 -> overflow/1
  Real-Imag to Complex/1 -> data_out/1
  Constant Im/1 -> Real-Imag to Complex/2
  Constant Re/1 -> Real-Imag to Complex/1

== system gm_dvbs2_stream_lib/AD936x Transmitter/Sink Variant/Terminator/SimCodegen Variant/CODEGEN ==
  data_in : Inport
  AD936x Transmitter : MATLABSystem  System=comm.SDRTxAD936x  IPAddress=192.168.3.2  uri=ip:10.0.0.200  CenterFrequencySource=Dialog  CenterFrequency=CenterFrequency  GainSource=Dialog  Gain=Gain  ChannelMapping=1  BasebandSampleRate=BasebandSampleRate  UnderflowOutputPort=off  ShowAdvancedProperties=off  UseCustomFilter=off  filtPathRates=filtPathRates  filtCoefficients=filtCoefficients  filtCoefficientSize=filtCoefficientSize  filtDecimInterpFactor=filtDecimInterpFactor  filtGain=filtGain  filtRFBandwidth=filtRFBandwidth  filterConfigStruct=filterConfigStruct  BypassUserLogic=off  DataSourceSelect=Input Port  DDSTone1Freq=DDSTone1Freq  DDSTone2Freq=DDSTone2Freq  DDSTone1Scale=DDSTone1Scale  DDSTone2Scale=DDSTone2Scale  DataTimeout=DataTimeout  ENSMPinControlMode=None  BISTLoopbackMode=Disabled  BISTToneInject=Disabled  BISTSignalGen=PRBS  BISTToneFreq=Fs/32  BISTToneLevel=0
      mask Type: comm.SDRTxAD936x
  wires:
  data_in/1 -> AD936x Transmitter/1

== system gm_dvbs2_stream_lib/AD936x Transmitter/Sink Variant/Terminator/SimCodegen Variant/SIM ==
  data_in : Inport
  Constant ov : Constant  Value=0  OutDataTypeStr=boolean
  Inherit Rate : socsharedlib_internal/Inherit Rate
  Terminator : Terminator
  underflow : Outport
  wires:
  Constant ov/1 -> Inherit Rate/1
  Inherit Rate/1 -> underflow/1
  data_in/1 -> Terminator/1, Inherit Rate/2
